simulink model "offset_rate210_20160802_144333"  (R2014a)
settings: Solver=FixedStepDiscrete  SolverMode=SingleTasking  StartTime=0.0  StopTime=10.0  FixedStep=0.002  RelTol=1e-3
settings Model: BufferReuse=off  Creator=yoshi12  LastModifiedBy=yoshi12
settings OptimizationCC: BlockReduction=off  OptimizeBlockIOStorage=off  BufferReuse=off  GlobalBufferReuse=off  ExpressionFolding=off  LocalBlockOutputs=off  OptimizeModelRefInitCode=on  LifeSpan=1  SimCompilerOptimization=off
settings DebuggingCC: MergeDetectMultiDrivingBlocksExec=error  MultiTaskRateTransMsg=warning  FrameProcessingCompatibilityMsg=error
settings RTWCC: SystemTargetFile=ert.tlc  GenCodeOnly=on  TemplateMakefile=ert_default_tmf  Description=Embedded Coder  GenerateReport=on  IncludeHyperlinkInReport=on  LaunchReport=on  GenerateTraceInfo=on  GenerateTraceReport=on  GenerateTraceReportSl=on  GenerateTraceReportSf=on  GenerateTraceReportEml=on  RTWCompilerOptimization=off
settings CodeAppCC: IgnoreCustomStorageClasses=off
settings ERTTargetCC: ParMdlRefBuildCompliant=on  CompOptLevelCompliant=on  ConcurrentExecutionCompliant=on  ERTFirstTimeCompliant=on  ModelStepFunctionPrototypeControlCompliant=on  CPPClassGenCompliant=on  InlinedParameterPlacement=Hierarchical  ERTCustomFileTemplate=example_file_process.tlc
settings ConfigComp: CovMetricSettings=dw  CovHtmlReporting=on  CovSaveCumulativeToWorkspaceVar=on  CovSaveSingleToWorkspaceVar=on  CovModelRefEnable=Off  CovExternalEMLEnable=off  CovSFcnEnable=off

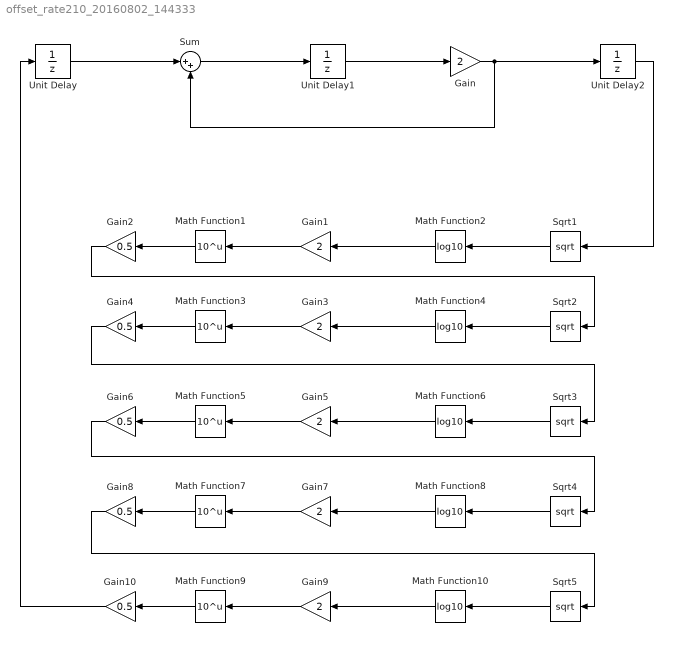
== system offset_rate210_20160802_144333 ==
  Gain : Gain  Gain=2  SampleTime=0.002
  Gain{1,3,5,7,9} (5 alike) : Gain  Gain=2  SampleTime=0.01
  Gain{2,4,6,8,10} (5 alike) : Gain  Gain=0.5  SampleTime=0.01
  Math Function{1,3,5,7,9} (5 alike) : Math  Operator=10^u  SampleTime=0.01  SaturateOnIntegerOverflow=on
  Math Function{2,4,6,8,10} (5 alike) : Math  Operator=log10  SampleTime=0.01  SaturateOnIntegerOverflow=on
  Sqrt{1..5} (5 alike) : Sqrt  SampleTime=0.01  SaturateOnIntegerOverflow=on
  Sum : Sum  Inputs=|++  SampleTime=0.002
  Unit Delay : UnitDelay  InitialCondition=1  SampleTime=-1
  Unit Delay1 : UnitDelay  InitialCondition=2  SampleTime=-1
  Unit Delay2 : UnitDelay  InitialCondition=1  SampleTime=-1
  wires:
  Unit Delay/1 -> Sum/1
  Sum/1 -> Unit Delay1/1
  Unit Delay1/1 -> Gain/1
  Gain/1 -> Sum/2, Unit Delay2/1
  Unit Delay2/1 -> Sqrt1/1
  Math Function3/1 -> Gain4/1
  Gain3/1 -> Math Function3/1
  Math Function4/1 -> Gain3/1
  Sqrt2/1 -> Math Function4/1
  Math Function5/1 -> Gain6/1
  Gain5/1 -> Math Function5/1
  Math Function6/1 -> Gain5/1
  Sqrt3/1 -> Math Function6/1
  Math Function7/1 -> Gain8/1
  Gain7/1 -> Math Function7/1
  Math Function8/1 -> Gain7/1
  Sqrt4/1 -> Math Function8/1
  Math Function9/1 -> Gain10/1
  Gain9/1 -> Math Function9/1
  Math Function10/1 -> Gain9/1
  Sqrt5/1 -> Math Function10/1
  Math Function1/1 -> Gain2/1
  Sqrt1/1 -> Math Function2/1
  Math Function2/1 -> Gain1/1
  Gain1/1 -> Math Function1/1
  Gain10/1 -> Unit Delay/1
  Gain2/1 -> Sqrt2/1
  Gain4/1 -> Sqrt3/1
  Gain6/1 -> Sqrt4/1
  Gain8/1 -> Sqrt5/1
